simulink model "testfcall_root_3"  (Simulink 8.2)
settings: Solver=FixedStepDiscrete  StartTime=0.0  StopTime=10.0  FixedStep=0.1  RelTol=1e-3
libraries: simulink x2
settings Model: Creator=smorikaw  LastModifiedBy=smorikaw
settings OptimizationCC: InlineParams=on
settings DebuggingCC: UnderspecifiedInitializationDetection=Simplified  FcnCallInpInsideContextMsg=EnableAllAsWarning
settings RTWCC: ProcessScript=grt_make_rtw_hook

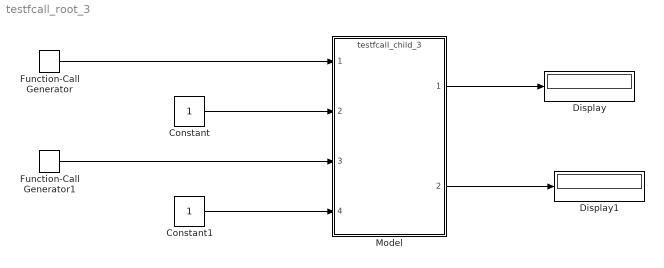
== system testfcall_root_3 ==
  Constant : Constant
  Constant1 : Constant
  Display : Display
  Display1 : Display
  Function-Call Generator : simulink/Ports & Subsystems/Function-Call Generator  sample_time=1  numberOfIterations=1
  Function-Call Generator1 : simulink/Ports & Subsystems/Function-Call Generator  sample_time=0.5  numberOfIterations=1
  Model : ModelReference  ModelNameDialog=testfcall_child_3  SimulationMode=Normal  ModelReferenceVersion=1.41  CopyOfModelName=testfcall_child_3  DefaultDataLogging=on
  wires:
  Model/1 -> Display/1
  Constant/1 -> Model/2
  Model/2 -> Display1/1
  Constant1/1 -> Model/4
  Function-Call Generator1/1 -> Model/3
  Function-Call Generator/1 -> Model/1
